simulink model "model_2_dq"  (R2021a)
settings: Solver=VariableStepAuto  StartTime=0.0  StopTime=0.5  FixedStep=1e-6  MaxStep=1e-4  RelTol=1e-4
values from neighbouring files (symbols this model uses):
  J = 0.0000048    (= 4.8e-06)    [BLDCParams.m]    (also in readSerial.m = 4.8e-05)
  Lsd = Ls    (= 0.0018)    [BLDCParams.m]    (also in readSerial.m)
  Lsd_Ldq = 0    [BLDCParams.m]    (also in readSerial.m)
  Lsq = Ls    (= 0.0018)    [BLDCParams.m]    (also in readSerial.m)
  Psi_f = Ke/Pole_pairs    (= 0.002375)    [BLDCParams.m]    (also in readSerial.m)
  refSpeed = 1500    [readSerial.m]
  Rs = 0.792/2    (= 0.396)    [BLDCParams.m]    (also in readSerial.m)
  Zp = Pole_pairs    (= 4)    [BLDCParams.m]    (also in readSerial.m)
libraries: pid_lib x3
settings Model: Creator=ba123  LastModifiedBy=worker
settings SolverCC: AlgebraicLoopSolver=TrustRegion
settings DataIOCC: ReturnWorkspaceOutputs=off
settings DebuggingCC: SFMachineParentedDataDiag=warning  ArithmeticOperatorsInVariantConditions=warning
settings SFSimCC: CustomCodeUndefinedFunction=UseInterfaceOnly

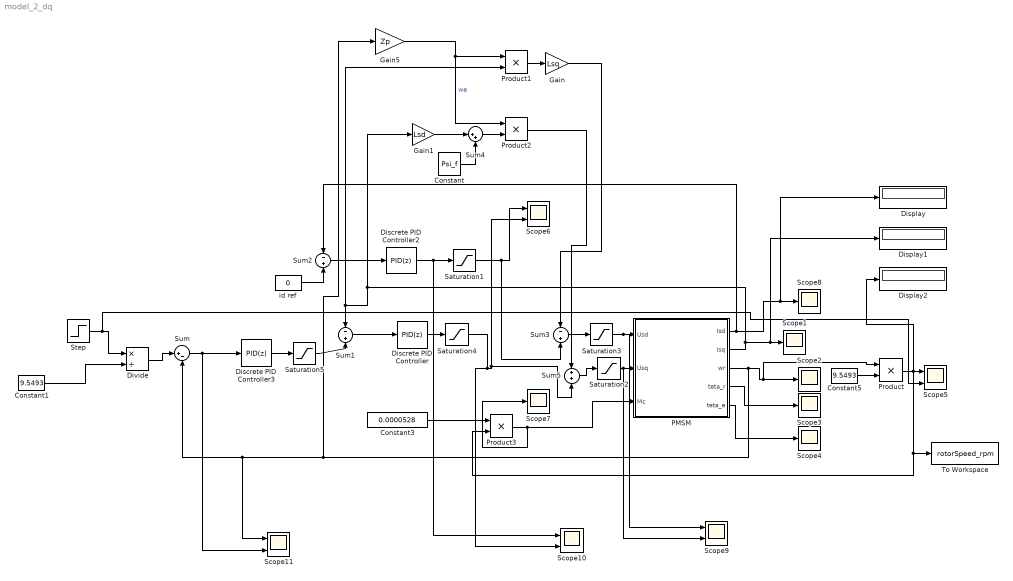
== system model_2_dq ==
  Constant : Constant  Value=Psi_f
  Constant1 : Constant  Value=9.5493
  Constant3 : Constant  Value=0.0000528
  Constant5 : Constant  Value=9.5493
  Discrete PID Controller : pid_lib/PID Controller  Controller=PID  Form=Parallel  TimeDomain=Discrete-time  UseExternalTs=off  SampleTime=1/16000  IntegratorMethod=Forward Euler  FilterMethod=Forward Euler  ControllerParametersSource=internal  P=100/16  I=40/256  D=0  UseFilter=on  N=2  TunerSelectOption=Transfer Function Based (PID Tuner App)  InitialConditionSource=internal  InitialConditionForIntegrator=0  InitialConditionForFilter=0  DifferentiatorICPrevScaledInput=0  ExternalReset=none  TrackingMode=off  Kt=1  LimitOutput=off  SatLimitsSource=internal  UpperSaturationLimit=inf  LowerSaturationLimit=-inf  LinearizeAsGain=off  AntiWindupMode=none  Kb=1  POutMin=[]  POutMax=[]  IOutMin=[]  IOutMax=[]  DOutMin=[]  DOutMax=[]  NOutMin=[]  NOutMax=[]  SumOutMin=[]  SumOutMax=[]  SaturationOutMin=[]  SaturationOutMax=[]  PParamMin=[]  PParamMax=[]  IParamMin=[]  IParamMax=[]  DParamMin=[]  DParamMax=[]  NParamMin=[]  NParamMax=[]  KbParamMin=[]  KbParamMax=[]  KtParamMin=[]  KtParamMax=[]  KbOutMin=[]  KbOutMax=[]  KtOutMin=[]  KtOutMax=[]  IntegratorOutMin=[]  IntegratorOutMax=[]  FilterOutMin=[]  FilterOutMax=[]  SumI1OutMin=[]  SumI1OutMax=[]  SumI2OutMin=[]  SumI2OutMax=[]  SumI3OutMin=[]  SumI3OutMax=[]  SumI4OutMin=[]  SumI4OutMax=[]  SumDOutMin=[]  SumDOutMax=[]  DifferentiatorOutMin=[]  DifferentiatorOutMax=[]  FilterDiffOutCoefMin=[]  FilterDiffOutCoefMax=[]  ReciprocalOutMin=[]  ReciprocalOutMax=[]  SumDenOutMin=[]  SumDenOutMax=[]  SumNumOutMin=[]  SumNumOutMax=[]  DivideOutMin=[]  DivideOutMax=[]  UdiffTsProdOutMin=[]  UdiffTsProdOutMax=[]  NTsProdOutMin=[]  NTsProdOutMax=[]  UintegralTsProdOutMin=[]  UintegralTsProdOutMax=[]  UngainTsProdOutMin=[]  UngainTsProdOutMax=[]  IntegratorContinuousStateAttributes=''  IntegratorStateMustResolveToSignalObject=off  IntegratorRTWStateStorageClass=Auto  FilterContinuousStateAttributes=''  FilterStateMustResolveToSignalObject=off  FilterRTWStateStorageClass=Auto  ParallelPVariant=InternalParameters  IdealPVariant=Disabled  IVariant=InternalParameters  DVariant=InternalParameters  IntegratorVariant=Discrete  SatVariant=Disabled  AWVariant=Passthrough  PCopyVariant=Disabled  TRVariant=Disabled  FdbkBlocksVariant=Forward  IdealPFdbkVariant=Disabled  SatFdbkVariant=Disabled  DerivativeFilterVariant=ForwardEulerFilter  NVariant=InternalParameters  NCopyVariant=Disabled  FilterICVariant=InternalICsFilter  IntegratorICVariant=InternalICs  ExternalResetVariant=Disabled  TRSumVariant=Passthrough  SumFdbkVariant=Disabled  SumVariant=Sum_PID  TsampFilterVariant=InternalTs  TsampNgainVariant=Passthrough  TsampIntegralVariant=Passthrough  ExternalSaturationOutDataTypeStr=Inherit: Same as second input
  Discrete PID Controller2 : pid_lib/PID Controller  Controller=PID  Form=Parallel  TimeDomain=Discrete-time  UseExternalTs=off  SampleTime=1/16000  IntegratorMethod=Forward Euler  FilterMethod=Forward Euler  ControllerParametersSource=internal  P=100/16  I=40/256  D=0  UseFilter=on  N=2  TunerSelectOption=Transfer Function Based (PID Tuner App)  InitialConditionSource=internal  InitialConditionForIntegrator=0  InitialConditionForFilter=0  DifferentiatorICPrevScaledInput=0  ExternalReset=none  TrackingMode=off  Kt=1  LimitOutput=off  SatLimitsSource=internal  UpperSaturationLimit=inf  LowerSaturationLimit=-inf  LinearizeAsGain=off  AntiWindupMode=none  Kb=1  POutMin=[]  POutMax=[]  IOutMin=[]  IOutMax=[]  DOutMin=[]  DOutMax=[]  NOutMin=[]  NOutMax=[]  SumOutMin=[]  SumOutMax=[]  SaturationOutMin=[]  SaturationOutMax=[]  PParamMin=[]  PParamMax=[]  IParamMin=[]  IParamMax=[]  DParamMin=[]  DParamMax=[]  NParamMin=[]  NParamMax=[]  KbParamMin=[]  KbParamMax=[]  KtParamMin=[]  KtParamMax=[]  KbOutMin=[]  KbOutMax=[]  KtOutMin=[]  KtOutMax=[]  IntegratorOutMin=[]  IntegratorOutMax=[]  FilterOutMin=[]  FilterOutMax=[]  SumI1OutMin=[]  SumI1OutMax=[]  SumI2OutMin=[]  SumI2OutMax=[]  SumI3OutMin=[]  SumI3OutMax=[]  SumI4OutMin=[]  SumI4OutMax=[]  SumDOutMin=[]  SumDOutMax=[]  DifferentiatorOutMin=[]  DifferentiatorOutMax=[]  FilterDiffOutCoefMin=[]  FilterDiffOutCoefMax=[]  ReciprocalOutMin=[]  ReciprocalOutMax=[]  SumDenOutMin=[]  SumDenOutMax=[]  SumNumOutMin=[]  SumNumOutMax=[]  DivideOutMin=[]  DivideOutMax=[]  UdiffTsProdOutMin=[]  UdiffTsProdOutMax=[]  NTsProdOutMin=[]  NTsProdOutMax=[]  UintegralTsProdOutMin=[]  UintegralTsProdOutMax=[]  UngainTsProdOutMin=[]  UngainTsProdOutMax=[]  IntegratorContinuousStateAttributes=''  IntegratorStateMustResolveToSignalObject=off  IntegratorRTWStateStorageClass=Auto  FilterContinuousStateAttributes=''  FilterStateMustResolveToSignalObject=off  FilterRTWStateStorageClass=Auto  ParallelPVariant=InternalParameters  IdealPVariant=Disabled  IVariant=InternalParameters  DVariant=InternalParameters  IntegratorVariant=Discrete  SatVariant=Disabled  AWVariant=Passthrough  PCopyVariant=Disabled  TRVariant=Disabled  FdbkBlocksVariant=Forward  IdealPFdbkVariant=Disabled  SatFdbkVariant=Disabled  DerivativeFilterVariant=ForwardEulerFilter  NVariant=InternalParameters  NCopyVariant=Disabled  FilterICVariant=InternalICsFilter  IntegratorICVariant=InternalICs  ExternalResetVariant=Disabled  TRSumVariant=Passthrough  SumFdbkVariant=Disabled  SumVariant=Sum_PID  TsampFilterVariant=InternalTs  TsampNgainVariant=Passthrough  TsampIntegralVariant=Passthrough  ExternalSaturationOutDataTypeStr=Inherit: Same as second input
  Discrete PID Controller3 : pid_lib/PID Controller  Controller=PID  Form=Parallel  TimeDomain=Discrete-time  UseExternalTs=off  SampleTime=1/16000  IntegratorMethod=Forward Euler  FilterMethod=Forward Euler  ControllerParametersSource=internal  P=250/1600  I=10/256*33  D=5/16000  UseFilter=on  N=2  TunerSelectOption=Transfer Function Based (PID Tuner App)  InitialConditionSource=internal  InitialConditionForIntegrator=0  InitialConditionForFilter=0  DifferentiatorICPrevScaledInput=0  ExternalReset=none  TrackingMode=off  Kt=1  LimitOutput=off  SatLimitsSource=internal  UpperSaturationLimit=inf  LowerSaturationLimit=-inf  LinearizeAsGain=off  AntiWindupMode=none  Kb=1  POutMin=[]  POutMax=[]  IOutMin=[]  IOutMax=[]  DOutMin=[]  DOutMax=[]  NOutMin=[]  NOutMax=[]  SumOutMin=[]  SumOutMax=[]  SaturationOutMin=[]  SaturationOutMax=[]  PParamMin=[]  PParamMax=[]  IParamMin=[]  IParamMax=[]  DParamMin=[]  DParamMax=[]  NParamMin=[]  NParamMax=[]  KbParamMin=[]  KbParamMax=[]  KtParamMin=[]  KtParamMax=[]  KbOutMin=[]  KbOutMax=[]  KtOutMin=[]  KtOutMax=[]  IntegratorOutMin=[]  IntegratorOutMax=[]  FilterOutMin=[]  FilterOutMax=[]  SumI1OutMin=[]  SumI1OutMax=[]  SumI2OutMin=[]  SumI2OutMax=[]  SumI3OutMin=[]  SumI3OutMax=[]  SumI4OutMin=[]  SumI4OutMax=[]  SumDOutMin=[]  SumDOutMax=[]  DifferentiatorOutMin=[]  DifferentiatorOutMax=[]  FilterDiffOutCoefMin=[]  FilterDiffOutCoefMax=[]  ReciprocalOutMin=[]  ReciprocalOutMax=[]  SumDenOutMin=[]  SumDenOutMax=[]  SumNumOutMin=[]  SumNumOutMax=[]  DivideOutMin=[]  DivideOutMax=[]  UdiffTsProdOutMin=[]  UdiffTsProdOutMax=[]  NTsProdOutMin=[]  NTsProdOutMax=[]  UintegralTsProdOutMin=[]  UintegralTsProdOutMax=[]  UngainTsProdOutMin=[]  UngainTsProdOutMax=[]  IntegratorContinuousStateAttributes=''  IntegratorStateMustResolveToSignalObject=off  IntegratorRTWStateStorageClass=Auto  FilterContinuousStateAttributes=''  FilterStateMustResolveToSignalObject=off  FilterRTWStateStorageClass=Auto  ParallelPVariant=InternalParameters  IdealPVariant=Disabled  IVariant=InternalParameters  DVariant=InternalParameters  IntegratorVariant=Discrete  SatVariant=Disabled  AWVariant=Passthrough  PCopyVariant=Disabled  TRVariant=Disabled  FdbkBlocksVariant=Forward  IdealPFdbkVariant=Disabled  SatFdbkVariant=Disabled  DerivativeFilterVariant=ForwardEulerFilter  NVariant=InternalParameters  NCopyVariant=Disabled  FilterICVariant=InternalICsFilter  IntegratorICVariant=InternalICs  ExternalResetVariant=Disabled  TRSumVariant=Passthrough  SumFdbkVariant=Disabled  SumVariant=Sum_PID  TsampFilterVariant=InternalTs  TsampNgainVariant=Passthrough  TsampIntegralVariant=Passthrough  ExternalSaturationOutDataTypeStr=Inherit: Same as second input
  Display : Display
  Display1 : Display
  Display2 : Display
  Divide : Product  Inputs=*/
  Gain : Gain  Gain=Lsq
  Gain1 : Gain  Gain=Lsd
  Gain5 : Gain  Gain=Zp
  "PMSM " : Subsystem
  Product{,1..3} (4 alike) : Product
  Saturation1 : Saturate  UpperLimit=10000  LowerLimit=-10000
  Saturation2 : Saturate  UpperLimit=24  LowerLimit=-24
  Saturation3 : Saturate  UpperLimit=24  LowerLimit=-24
  Saturation4 : Saturate  UpperLimit=10000  LowerLimit=-10000
  Saturation5 : Saturate  UpperLimit=10000  LowerLimit=-10000
  Scope{1..4,7..8} (6 alike) : Scope
  Scope{5..6,9..11} (5 alike) : Scope  NumInputPorts=2
  Step : Step  Time=0  After=refSpeed  SampleTime=0
  Sum : Sum  Inputs=|+-
  Sum1 : Sum  Inputs=-+
  Sum2 : Sum  Inputs=-+
  Sum3 : Sum  Inputs=-+
  Sum4 : Sum  Inputs=|++
  Sum5 : Sum
  To Workspace : ToWorkspace  VariableName=rotorSpeed_rpm  SaveFormat=Structure With Time  SampleTime=-1
  id ref : Constant  Value=0
  wires:
  "PMSM "/1(Isd) -> Display/1, Scope8/1, Sum2/1
  "PMSM "/5(teta_e) -> Scope4/1
  Constant5/1 -> Product/2
  Product/1 -> Product3/2, To Workspace/1, Display2/1, Scope5/1
  id ref/1 -> Sum2/2
  Constant1/1 -> Divide/2
  Divide/1 -> Sum/1
  "PMSM "/4(teta_r) -> Scope3/1
  "PMSM "/3(wr) -> Gain5/1, Scope11/1, Sum/2, Product/1, Scope2/1
  Step/1 -> Scope5/2, Divide/1
  Product1/1 -> Gain/1
  Gain/1 -> Sum3/1
  Sum3/1 -> Saturation3/1
  Sum4/1 -> Product2/2
  Constant/1 -> Sum4/2
  "PMSM "/2(Isq) -> Display1/1, Scope1/1, Product1/2, Sum1/1, Gain1/1
  Gain1/1 -> Sum4/1
  Gain5/1 -> Product2/1, Product1/1  "we"
  Product2/1 -> Sum5/1
  Discrete PID Controller2/1 -> Scope10/1, Saturation1/1
  Saturation3/1 -> Scope9/1, "PMSM "/1(Usd)
  Sum5/1 -> Saturation2/1
  Saturation2/1 -> Scope9/2, "PMSM "/2(Usq)
  Constant3/1 -> Product3/1
  Product3/1 -> Scope7/1, "PMSM "/3(Mc)
  Discrete PID Controller/1 -> Saturation4/1
  Discrete PID Controller3/1 -> Saturation5/1
  Saturation5/1 -> Sum1/2
  Sum/1 -> Scope11/2, Discrete PID Controller3/1
  Sum2/1 -> Discrete PID Controller2/1
  Sum1/1 -> Discrete PID Controller/1
  Saturation1/1 -> Scope6/1, Sum3/2
  Saturation4/1 -> Scope10/2, Sum5/2, Scope6/2

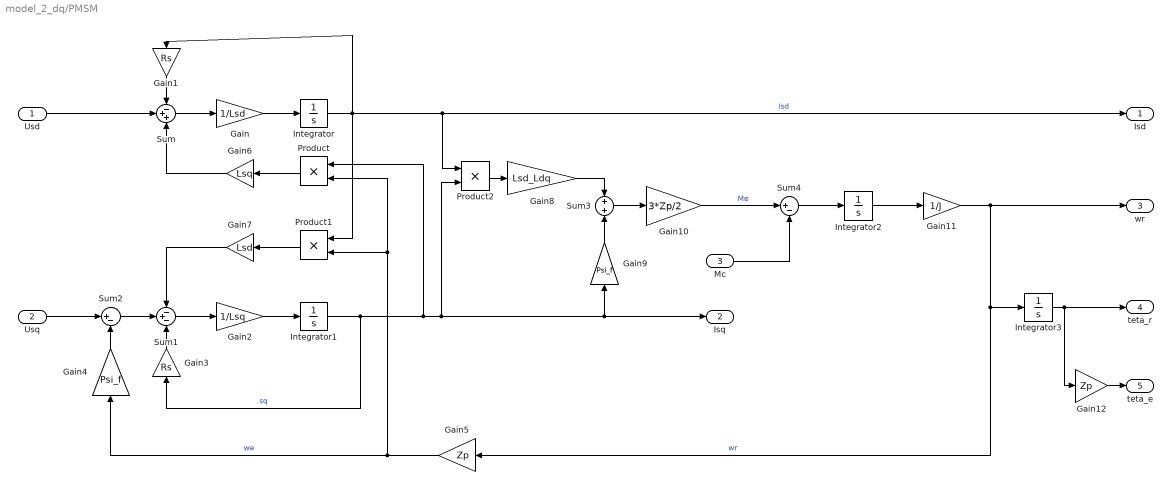
== system model_2_dq/PMSM  ==
  Usd : Inport
  Usq : Inport  Port=2
  Mc : Inport  Port=3
  Gain : Gain  Gain=1/Lsd
  Gain1 : Gain  Gain=Rs
  Gain10 : Gain  Gain=3*Zp/2
  Gain11 : Gain  Gain=1/J
  Gain12 : Gain  Gain=Zp
  Gain2 : Gain  Gain=1/Lsq
  Gain3 : Gain  Gain=Rs
  Gain4 : Gain  Gain=Psi_f
  Gain5 : Gain  Gain=Zp
  Gain6 : Gain  Gain=Lsq
  Gain7 : Gain  Gain=Lsd
  Gain8 : Gain  Gain=Lsd_Ldq
  Gain9 : Gain  Gain=Psi_f
  Integrator{,1..3} (4 alike) : Integrator
  Product : Product
  Product1 : Product
  Product2 : Product
  Sum : Sum  Inputs=-++
  Sum1 : Sum  Inputs=-+-
  Sum2 : Sum  Inputs=|+-
  Sum3 : Sum
  Sum4 : Sum  Inputs=|+-
  Isd : Outport  VectorParamsAs1DForOutWhenUnconnected=off
  Isq : Outport  Port=2  VectorParamsAs1DForOutWhenUnconnected=off
  wr : Outport  Port=3  VectorParamsAs1DForOutWhenUnconnected=off
  teta_r : Outport  Port=4  VectorParamsAs1DForOutWhenUnconnected=off
  teta_e : Outport  Port=5  VectorParamsAs1DForOutWhenUnconnected=off
  wires:
  Gain/1 -> Integrator/1
  Sum/1 -> Gain/1
  Gain1/1 -> Sum/1
  Usd/1 -> Sum/2
  Gain2/1 -> Integrator1/1
  Sum1/1 -> Gain2/1
  Gain3/1 -> Sum1/3
  Sum2/1 -> Sum1/2
  Usq/1 -> Sum2/1
  Gain4/1 -> Sum2/2
  Gain5/1 -> Product/2, Product1/2, Gain4/1  "we"
  Product/1 -> Gain6/1
  Gain6/1 -> Sum/3
  Integrator1/1 -> Product/1, Isq/1, Gain9/1, Product2/2, Gain3/1  "sq"
  Integrator/1 -> Gain1/1, Isd/1, Product2/1, Product1/1  "Isd"
  Gain7/1 -> Sum1/1
  Product1/1 -> Gain7/1
  Product2/1 -> Gain8/1
  Gain8/1 -> Sum3/1
  Gain9/1 -> Sum3/2
  Sum3/1 -> Gain10/1
  Gain10/1 -> Sum4/1  "Me"
  Gain11/1 -> wr/1, Integrator3/1, Gain5/1  "wr"
  Sum4/1 -> Integrator2/1
  Integrator2/1 -> Gain11/1
  Mc/1 -> Sum4/2
  Integrator3/1 -> Gain12/1, teta_r/1
  Gain12/1 -> teta_e/1
